simulink model "ModeStEnCtrl6s7s"  (R2024b)
settings: Solver=FixedStepDiscrete  StartTime=0.0  StopTime=10.0  FixedStep=0.01  RelTol=1e-3
undefined symbols (not defined in the file or in its folder): BigFour6sStEnCtrl_Cal, BigFourStEnCtrl_Cal, ComfortMdLStEnCtrl_Cal, ComfortMdRStEnCtrl_Cal, EZE5576sStEnCtrl_Cal, EZE557StEnCtrl_Cal, EZQStEnCtrl_Cal, FirstTrig, INTMLStEnCtrl_Cal, INTMRStEnCtrl_Cal, KeSMSuVehicleModelConfig_Val, LugL6sStEnCtrl_Cal, LugL7sStEnCtrl_Cal, LugR6sStEnCtrl_Cal, LugR7sStEnCtrl_Cal, Md27StEnCtrl_Cal, Md28StEnCtrl_Cal, Md30StEnCtrl_Cal, Md31StEnCtrl_Cal, Md32StEnCtrl_Cal, Md53StEnCtrl_Cal, Md57StEnCtrl_Cal, Md58StEnCtrl_Cal, Md58TrgtPos_Set, Md61StEnCtrl_Cal, Md62StEnCtrl_Cal, RecvR4sStEnCtrl_Cal, VIPL557LTStEnCtrl_Cal, VIPL557StEnCtrl_Cal, VIPLExit557StEnCtrl_Cal, VIPLExit557TrgtPos_Set, VIPR557LTStEnCtrl_Cal, VIPR557StEnCtrl_Cal, VIPRExit557StEnCtrl_Cal, VIPRExit557TrgtPos_Set
libraries: simulink x30
(part 1 of 2)
settings Model: Creator=sn2xws  LastModifiedBy=sn55gm
settings Model: ModifiedHistory=|
  | 2024.5.8
  | V3.0.0 557 eze 及复位模式变更
  | 2024.7.9
  | V3.0.1 557 模式流程V1.9
  | V3.0.2 md30 md31 md32 md53增加mdfirsttrig
  | V3.0.3 md1增加firsttrig
  | V3.0.4 智享增加FirstTrig
  | V3.0.5 Md28 FirstTrig信号遗漏连接
  | V3.0.6 Md27 FirstTrig信号遗漏连接
  | V3.0.7 Md8,Md9增加FirstTrig信号
  | V3.0.8 新增Md56
  | V3.0.9 新增Md57，Md58
  | V3.1.0 BUG 969014 Lug7sRStEnCtrl en 属性改为reset
  | V3.13.0 新增Md61 md62
settings SolverCC: AlgebraicLoopSolver=TrustRegion
settings DataIOCC: SaveFormat=StructureWithTime  ReturnWorkspaceOutputs=off
settings OptimizationCC: DefaultParameterBehavior=Inlined  EnhancedBackFolding=on  PassReuseOutputArgsAs=Individual arguments  ZeroExternalMemoryAtStartup=off  ZeroInternalMemoryAtStartup=off  OptimizeBlockOrder=speed  DifferentSizesBufferReuse=on  OptimizationCustomize=off  EfficientTunableParamExpr=on
settings DebuggingCC: ParameterTunabilityLossMsg=error  UnconnectedInputMsg=warning  UnconnectedOutputMsg=warning  UnconnectedLineMsg=warning  ArithmeticOperatorsInVariantConditions=warning
settings ModelReferenceCC: EnableRefExpFcnMdlSchedulingChecks=on
settings SFSimCC: MATLABDynamicMemAlloc=off  CustomCodeUndefinedFunction=UseInterfaceOnly
settings RTWCC: Description=AUTOSAR  SystemTargetFile=autosar.tlc  GenCodeOnly=on  TemplateMakefile=ert_default_tmf  GenerateReport=on  IncludeHyperlinkInReport=on  LaunchReport=on  DataTypeReplacement=CDataTypesFixedWidth  GenerateTraceInfo=on  GenerateTraceReport=on  GenerateTraceReportSl=on  GenerateTraceReportSf=on  GenerateTraceReportEml=on  GenerateCodeMetricsReport=on  GPUComputeCapability=3.5
settings CodeAppCC: ForceParamTrailComments=on  IgnoreCustomStorageClasses=off  OperatorAnnotations=on  SimulinkDataObjDesc=on  SFDataObjDesc=on  InsertBlockDesc=on
settings STFCustomTargetCC: TargetLangStandard=C99 (ISO)  MultiwordLength=256  ParMdlRefBuildCompliant=on  CompOptLevelCompliant=on  IncludeMdlTerminateFcn=off  CombineOutputUpdateFcns=on  SuppressErrorStatus=on  ERTCustomFileBanners=on  SupportNonFinite=off  SupportComplex=off  SupportContinuousTime=off  SupportNonInlinedSFcns=off  RemoveResetFunc=on  MATLABClassNameForMDSCustomization=Simulink.SoftwareTarget.ERTCustomization  AutosarCompliant=on  UseToolchainInfoCompliant=on  LookupTableObjectStructAxisOrder=2,1,3,4,...  LUTObjectStructOrderEvenSpacing=Size,Table,Breakpoints  SystemTargetFile=autosar.tlc
settings ERTTargetCC: TargetLangStandard=C99 (ISO)  ConcurrentExecutionCompliant=off  IncludeMdlTerminateFcn=off  SuppressErrorStatus=on  SupportNonFinite=off  SupportComplex=off  ModelStepFunctionPrototypeControlCompliant=off  CPPClassGenCompliant=off  AutosarCompliant=on  LookupTableObjectStructAxisOrder=2,1,3,4,...  LUTObjectStructOrderEvenSpacing=Size,Table,Breakpoints  ERTCustomFileTemplate=example_file_process.tlc  ERTFilePackagingFormat=Compact  BooleanTrueId=TRUE  BooleanFalseId=FALSE  DynamicArrayContainerType=coder::array

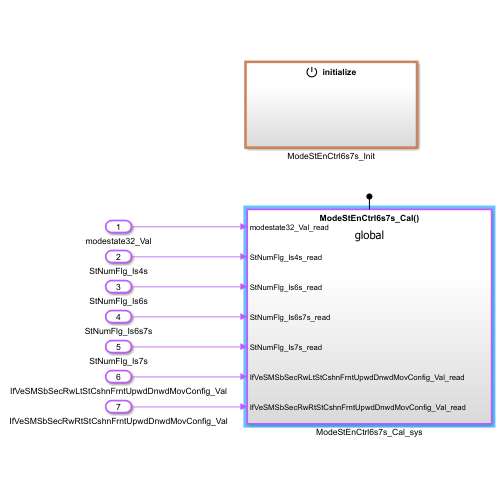
[thumbnail: Simulink's stored preview of the top-level diagram]
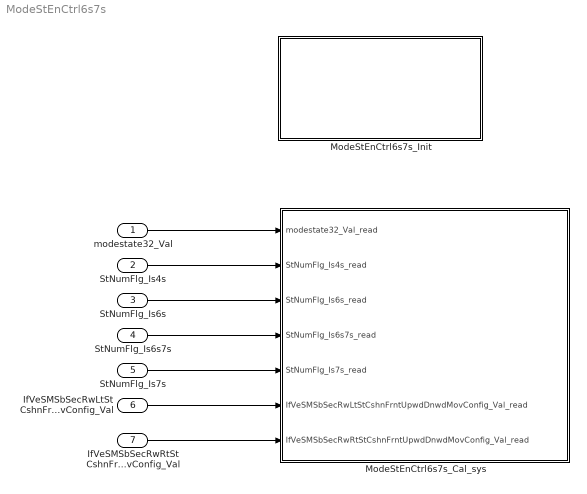
== system ModeStEnCtrl6s7s ==
  modestate32_Val : Inport  OutDataTypeStr=uint32  PortDimensions=1
  StNumFlg_Is4s : Inport  Port=2  OutDataTypeStr=boolean  PortDimensions=1
  StNumFlg_Is6s : Inport  Port=3  OutDataTypeStr=boolean  PortDimensions=1
  StNumFlg_Is6s7s : Inport  Port=4  OutDataTypeStr=boolean  PortDimensions=1
  StNumFlg_Is7s : Inport  Port=5  OutDataTypeStr=boolean  PortDimensions=1
  IfVeSMSbSecRwLtStCshnFrntUpwdDnwdMovConfig_Val : Inport  Port=6  OutDataTypeStr=boolean  PortDimensions=1
  IfVeSMSbSecRwRtStCshnFrntUpwdDnwdMovConfig_Val : Inport  Port=7  OutDataTypeStr=boolean  PortDimensions=1
  ModeStEnCtrl6s7s_Cal_sys : Subsystem
  ModeStEnCtrl6s7s_Init : Subsystem
  wires:
  modestate32_Val/1 -> ModeStEnCtrl6s7s_Cal_sys/1(modestate32_Val_read)
  StNumFlg_Is4s/1 -> ModeStEnCtrl6s7s_Cal_sys/2(StNumFlg_Is4s_read)
  StNumFlg_Is6s/1 -> ModeStEnCtrl6s7s_Cal_sys/3(StNumFlg_Is6s_read)
  StNumFlg_Is6s7s/1 -> ModeStEnCtrl6s7s_Cal_sys/4(StNumFlg_Is6s7s_read)
  StNumFlg_Is7s/1 -> ModeStEnCtrl6s7s_Cal_sys/5(StNumFlg_Is7s_read)
  IfVeSMSbSecRwLtStCshnFrntUpwdDnwdMovConfig_Val/1 -> ModeStEnCtrl6s7s_Cal_sys/6(IfVeSMSbSecRwLtStCshnFrntUpwdDnwdMovConfig_Val_read)
  IfVeSMSbSecRwRtStCshnFrntUpwdDnwdMovConfig_Val/1 -> ModeStEnCtrl6s7s_Cal_sys/7(IfVeSMSbSecRwRtStCshnFrntUpwdDnwdMovConfig_Val_read)

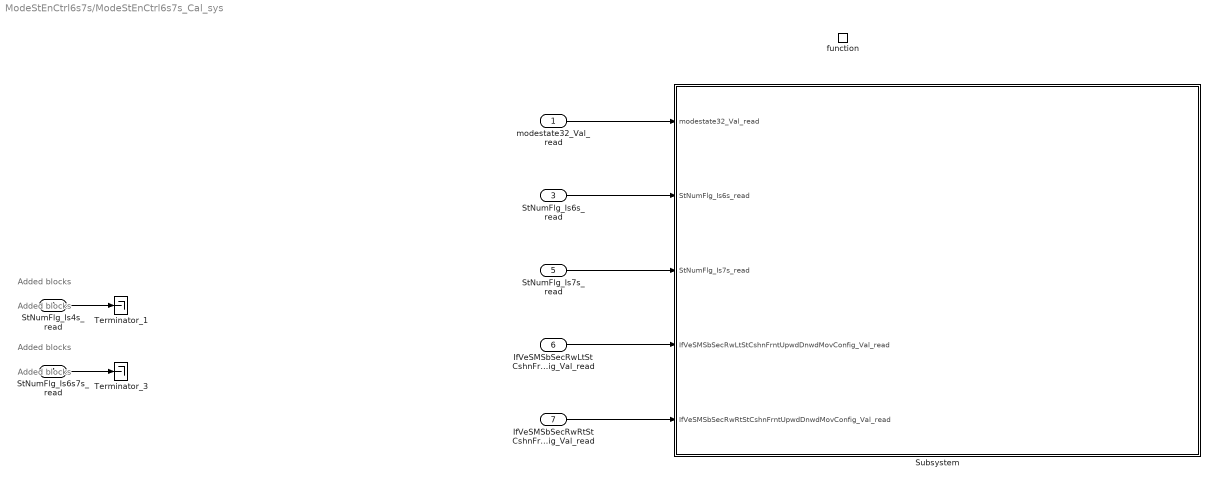
== system ModeStEnCtrl6s7s/ModeStEnCtrl6s7s_Cal_sys ==
  note: Added blocks
  note: Added blocks
  note: Added blocks
  note: Added blocks
  modestate32_Val_read : Inport
  StNumFlg_Is4s_read : Inport  Port=2
  StNumFlg_Is6s_read : Inport  Port=3
  StNumFlg_Is6s7s_read : Inport  Port=4
  StNumFlg_Is7s_read : Inport  Port=5
  IfVeSMSbSecRwLtStCshnFrntUpwdDnwdMovConfig_Val_read : Inport  Port=6
  IfVeSMSbSecRwRtStCshnFrntUpwdDnwdMovConfig_Val_read : Inport  Port=7
  function : TriggerPort  TriggerType=function-call  IsSimulinkFunction=on  FunctionName=ModeStEnCtrl6s7s_Cal  VariantControl=(inherit)
  Subsystem : Subsystem
  Terminator_1 : Terminator
  Terminator_3 : Terminator
  wires:
  modestate32_Val_read/1 -> Subsystem/1(modestate32_Val_read)
  StNumFlg_Is4s_read/1 -> Terminator_1/1
  StNumFlg_Is6s7s_read/1 -> Terminator_3/1
  StNumFlg_Is7s_read/1 -> Subsystem/3(StNumFlg_Is7s_read)
  StNumFlg_Is6s_read/1 -> Subsystem/2(StNumFlg_Is6s_read)
  IfVeSMSbSecRwLtStCshnFrntUpwdDnwdMovConfig_Val_read/1 -> Subsystem/4(IfVeSMSbSecRwLtStCshnFrntUpwdDnwdMovConfig_Val_read)
  IfVeSMSbSecRwRtStCshnFrntUpwdDnwdMovConfig_Val_read/1 -> Subsystem/5(IfVeSMSbSecRwRtStCshnFrntUpwdDnwdMovConfig_Val_read)

== system ModeStEnCtrl6s7s/ModeStEnCtrl6s7s_Init ==
  note: Added blocks
  Event Listener : EventListener  EventName=reset
  PA_KeSMSuVehicleModelConfig_Val : Constant  Value=KeSMSuVehicleModelConfig_Val
  Terminator_1 : Terminator
  wires:
  PA_KeSMSuVehicleModelConfig_Val/1 -> Terminator_1/1

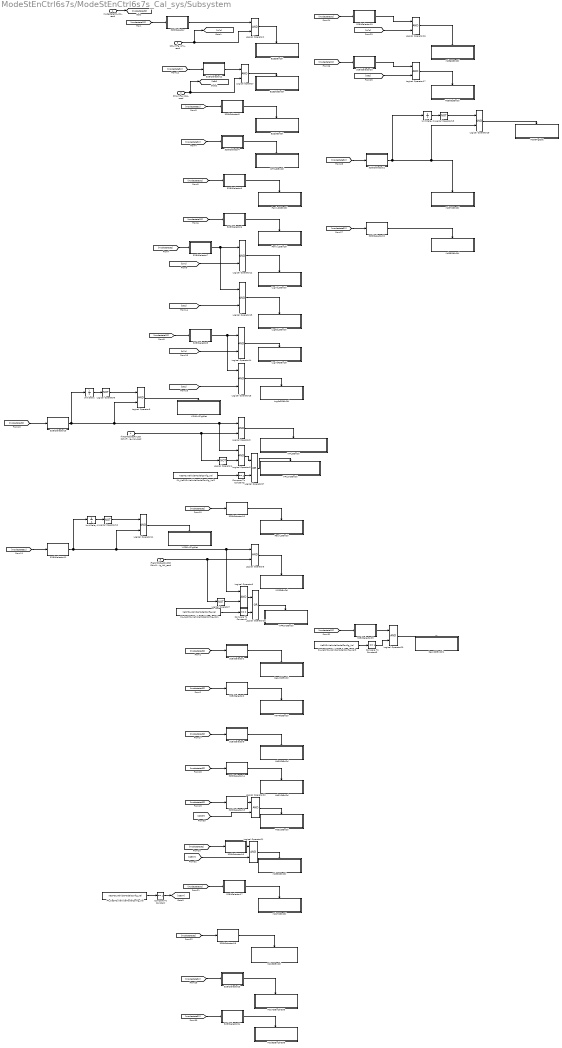
== system ModeStEnCtrl6s7s/ModeStEnCtrl6s7s_Cal_sys/Subsystem ==
  modestate32_Val_read : Inport
  StNumFlg_Is6s_read : Inport  Port=2
  StNumFlg_Is7s_read : Inport  Port=3
  IfVeSMSbSecRwLtStCshnFrntUpwdDnwdMovConfig_Val_read : Inport  Port=4
  IfVeSMSbSecRwRtStCshnFrntUpwdDnwdMovConfig_Val_read : Inport  Port=5
  32BitSelector : Subsystem  mask(32 Bit Selector){BitNum=0}
      mask prompts: BitNum "Select Bit Number"
      mask help: Allows selection of a particular bit (0-31) out of a packed word up to 32 bits long. Output will be true if the bit number selected via the mask parameter is equal to one.
      mask TypeOptions BitNum: 0 | 1 | 2 | 3 | 4 | 5 | 6 | 7 | 8 | 9 | 10 | 11 | 12 | 13 | 14 | 15 | 16 | 17 | 18 | 19 | 20 | 21 | 22 | 23 | 24 | 25 | 26 | 27 | 28 | 29 | 30 | 31
      mask Display:
      | text(0.5, 0.8,'BIT','horizontalAlignment','center')
      | text(0.5, 0.5,'SELECTOR','horizontalAlignment','center')
      | text(0.5, 0.2,['-- Bit ',char(get_param(gcb,'BitNum')),' --'],'horizontalAlignment','center')
  32BitSelector1 : Subsystem  mask(32 Bit Selector){BitNum=12}
      mask prompts: BitNum "Select Bit Number"
      mask help: Allows selection of a particular bit (0-31) out of a packed word up to 32 bits long. Output will be true if the bit number selected via the mask parameter is equal to one.
      mask TypeOptions BitNum: 0 | 1 | 2 | 3 | 4 | 5 | 6 | 7 | 8 | 9 | 10 | 11 | 12 | 13 | 14 | 15 | 16 | 17 | 18 | 19 | 20 | 21 | 22 | 23 | 24 | 25 | 26 | 27 | 28 | 29 | 30 | 31
      mask Display:
      | text(0.5, 0.8,'BIT','horizontalAlignment','center')
      | text(0.5, 0.5,'SELECTOR','horizontalAlignment','center')
      | text(0.5, 0.2,['-- Bit ',char(get_param(gcb,'BitNum')),' --'],'horizontalAlignment','center')
  32BitSelector10 : Subsystem  mask(32 Bit Selector){BitNum=10}
      mask prompts: BitNum "Select Bit Number"
      mask help: Allows selection of a particular bit (0-31) out of a packed word up to 32 bits long. Output will be true if the bit number selected via the mask parameter is equal to one.
      mask TypeOptions BitNum: 0 | 1 | 2 | 3 | 4 | 5 | 6 | 7 | 8 | 9 | 10 | 11 | 12 | 13 | 14 | 15 | 16 | 17 | 18 | 19 | 20 | 21 | 22 | 23 | 24 | 25 | 26 | 27 | 28 | 29 | 30 | 31
      mask Display:
      | text(0.5, 0.8,'BIT','horizontalAlignment','center')
      | text(0.5, 0.5,'SELECTOR','horizontalAlignment','center')
      | text(0.5, 0.2,['-- Bit ',char(get_param(gcb,'BitNum')),' --'],'horizontalAlignment','center')
  32BitSelector11 : Subsystem  mask(32 Bit Selector){BitNum=11}
      mask prompts: BitNum "Select Bit Number"
      mask help: Allows selection of a particular bit (0-31) out of a packed word up to 32 bits long. Output will be true if the bit number selected via the mask parameter is equal to one.
      mask TypeOptions BitNum: 0 | 1 | 2 | 3 | 4 | 5 | 6 | 7 | 8 | 9 | 10 | 11 | 12 | 13 | 14 | 15 | 16 | 17 | 18 | 19 | 20 | 21 | 22 | 23 | 24 | 25 | 26 | 27 | 28 | 29 | 30 | 31
      mask Display:
      | text(0.5, 0.8,'BIT','horizontalAlignment','center')
      | text(0.5, 0.5,'SELECTOR','horizontalAlignment','center')
      | text(0.5, 0.2,['-- Bit ',char(get_param(gcb,'BitNum')),' --'],'horizontalAlignment','center')
  32BitSelector12 : Subsystem  mask(32 Bit Selector){BitNum=0}
      mask prompts: BitNum "Select Bit Number"
      mask help: Allows selection of a particular bit (0-31) out of a packed word up to 32 bits long. Output will be true if the bit number selected via the mask parameter is equal to one.
      mask TypeOptions BitNum: 0 | 1 | 2 | 3 | 4 | 5 | 6 | 7 | 8 | 9 | 10 | 11 | 12 | 13 | 14 | 15 | 16 | 17 | 18 | 19 | 20 | 21 | 22 | 23 | 24 | 25 | 26 | 27 | 28 | 29 | 30 | 31
      mask Display:
      | text(0.5, 0.8,'BIT','horizontalAlignment','center')
      | text(0.5, 0.5,'SELECTOR','horizontalAlignment','center')
      | text(0.5, 0.2,['-- Bit ',char(get_param(gcb,'BitNum')),' --'],'horizontalAlignment','center')
  32BitSelector13 : Subsystem  mask(32 Bit Selector){BitNum=9}
      mask prompts: BitNum "Select Bit Number"
      mask help: Allows selection of a particular bit (0-31) out of a packed word up to 32 bits long. Output will be true if the bit number selected via the mask parameter is equal to one.
      mask TypeOptions BitNum: 0 | 1 | 2 | 3 | 4 | 5 | 6 | 7 | 8 | 9 | 10 | 11 | 12 | 13 | 14 | 15 | 16 | 17 | 18 | 19 | 20 | 21 | 22 | 23 | 24 | 25 | 26 | 27 | 28 | 29 | 30 | 31
      mask Display:
      | text(0.5, 0.8,'BIT','horizontalAlignment','center')
      | text(0.5, 0.5,'SELECTOR','horizontalAlignment','center')
      | text(0.5, 0.2,['-- Bit ',char(get_param(gcb,'BitNum')),' --'],'horizontalAlignment','center')
  32BitSelector14 : Subsystem  mask(32 Bit Selector){BitNum=30}
      mask prompts: BitNum "Select Bit Number"
      mask help: Allows selection of a particular bit (0-31) out of a packed word up to 32 bits long. Output will be true if the bit number selected via the mask parameter is equal to one.
      mask TypeOptions BitNum: 0 | 1 | 2 | 3 | 4 | 5 | 6 | 7 | 8 | 9 | 10 | 11 | 12 | 13 | 14 | 15 | 16 | 17 | 18 | 19 | 20 | 21 | 22 | 23 | 24 | 25 | 26 | 27 | 28 | 29 | 30 | 31
      mask Display:
      | text(0.5, 0.8,'BIT','horizontalAlignment','center')
      | text(0.5, 0.5,'SELECTOR','horizontalAlignment','center')
      | text(0.5, 0.2,['-- Bit ',char(get_param(gcb,'BitNum')),' --'],'horizontalAlignment','center')
  32BitSelector15 : Subsystem  mask(32 Bit Selector){BitNum=31}
      mask prompts: BitNum "Select Bit Number"
      mask help: Allows selection of a particular bit (0-31) out of a packed word up to 32 bits long. Output will be true if the bit number selected via the mask parameter is equal to one.
      mask TypeOptions BitNum: 0 | 1 | 2 | 3 | 4 | 5 | 6 | 7 | 8 | 9 | 10 | 11 | 12 | 13 | 14 | 15 | 16 | 17 | 18 | 19 | 20 | 21 | 22 | 23 | 24 | 25 | 26 | 27 | 28 | 29 | 30 | 31
      mask Display:
      | text(0.5, 0.8,'BIT','horizontalAlignment','center')
      | text(0.5, 0.5,'SELECTOR','horizontalAlignment','center')
      | text(0.5, 0.2,['-- Bit ',char(get_param(gcb,'BitNum')),' --'],'horizontalAlignment','center')
  32BitSelector16 : Subsystem  mask(32 Bit Selector){BitNum=17}
      mask prompts: BitNum "Select Bit Number"
      mask help: Allows selection of a particular bit (0-31) out of a packed word up to 32 bits long. Output will be true if the bit number selected via the mask parameter is equal to one.
      mask TypeOptions BitNum: 0 | 1 | 2 | 3 | 4 | 5 | 6 | 7 | 8 | 9 | 10 | 11 | 12 | 13 | 14 | 15 | 16 | 17 | 18 | 19 | 20 | 21 | 22 | 23 | 24 | 25 | 26 | 27 | 28 | 29 | 30 | 31
      mask Display:
      | text(0.5, 0.8,'BIT','horizontalAlignment','center')
      | text(0.5, 0.5,'SELECTOR','horizontalAlignment','center')
      | text(0.5, 0.2,['-- Bit ',char(get_param(gcb,'BitNum')),' --'],'horizontalAlignment','center')
  32BitSelector17 : Subsystem  mask(32 Bit Selector){BitNum=26}
      mask prompts: BitNum "Select Bit Number"
      mask help: Allows selection of a particular bit (0-31) out of a packed word up to 32 bits long. Output will be true if the bit number selected via the mask parameter is equal to one.
      mask TypeOptions BitNum: 0 | 1 | 2 | 3 | 4 | 5 | 6 | 7 | 8 | 9 | 10 | 11 | 12 | 13 | 14 | 15 | 16 | 17 | 18 | 19 | 20 | 21 | 22 | 23 | 24 | 25 | 26 | 27 | 28 | 29 | 30 | 31
      mask Display:
      | text(0.5, 0.8,'BIT','horizontalAlignment','center')
      | text(0.5, 0.5,'SELECTOR','horizontalAlignment','center')
      | text(0.5, 0.2,['-- Bit ',char(get_param(gcb,'BitNum')),' --'],'horizontalAlignment','center')
  32BitSelector18 : Subsystem  mask(32 Bit Selector){BitNum=27}
      mask prompts: BitNum "Select Bit Number"
      mask help: Allows selection of a particular bit (0-31) out of a packed word up to 32 bits long. Output will be true if the bit number selected via the mask parameter is equal to one.
      mask TypeOptions BitNum: 0 | 1 | 2 | 3 | 4 | 5 | 6 | 7 | 8 | 9 | 10 | 11 | 12 | 13 | 14 | 15 | 16 | 17 | 18 | 19 | 20 | 21 | 22 | 23 | 24 | 25 | 26 | 27 | 28 | 29 | 30 | 31
      mask Display:
      | text(0.5, 0.8,'BIT','horizontalAlignment','center')
      | text(0.5, 0.5,'SELECTOR','horizontalAlignment','center')
      | text(0.5, 0.2,['-- Bit ',char(get_param(gcb,'BitNum')),' --'],'horizontalAlignment','center')
  32BitSelector19 : Subsystem  mask(32 Bit Selector){BitNum=24}
      mask prompts: BitNum "Select Bit Number"
      mask help: Allows selection of a particular bit (0-31) out of a packed word up to 32 bits long. Output will be true if the bit number selected via the mask parameter is equal to one.
      mask TypeOptions BitNum: 0 | 1 | 2 | 3 | 4 | 5 | 6 | 7 | 8 | 9 | 10 | 11 | 12 | 13 | 14 | 15 | 16 | 17 | 18 | 19 | 20 | 21 | 22 | 23 | 24 | 25 | 26 | 27 | 28 | 29 | 30 | 31
      mask Display:
      | text(0.5, 0.8,'BIT','horizontalAlignment','center')
      | text(0.5, 0.5,'SELECTOR','horizontalAlignment','center')
      | text(0.5, 0.2,['-- Bit ',char(get_param(gcb,'BitNum')),' --'],'horizontalAlignment','center')
  32BitSelector2 : Subsystem  mask(32 Bit Selector){BitNum=19}
      mask prompts: BitNum "Select Bit Number"
      mask help: Allows selection of a particular bit (0-31) out of a packed word up to 32 bits long. Output will be true if the bit number selected via the mask parameter is equal to one.
      mask TypeOptions BitNum: 0 | 1 | 2 | 3 | 4 | 5 | 6 | 7 | 8 | 9 | 10 | 11 | 12 | 13 | 14 | 15 | 16 | 17 | 18 | 19 | 20 | 21 | 22 | 23 | 24 | 25 | 26 | 27 | 28 | 29 | 30 | 31
      mask Display:
      | text(0.5, 0.8,'BIT','horizontalAlignment','center')
      | text(0.5, 0.5,'SELECTOR','horizontalAlignment','center')
      | text(0.5, 0.2,['-- Bit ',char(get_param(gcb,'BitNum')),' --'],'horizontalAlignment','center')
  32BitSelector20 : Subsystem  mask(32 Bit Selector){BitNum=24}
      mask prompts: BitNum "Select Bit Number"
      mask help: Allows selection of a particular bit (0-31) out of a packed word up to 32 bits long. Output will be true if the bit number selected via the mask parameter is equal to one.
      mask TypeOptions BitNum: 0 | 1 | 2 | 3 | 4 | 5 | 6 | 7 | 8 | 9 | 10 | 11 | 12 | 13 | 14 | 15 | 16 | 17 | 18 | 19 | 20 | 21 | 22 | 23 | 24 | 25 | 26 | 27 | 28 | 29 | 30 | 31
      mask Display:
      | text(0.5, 0.8,'BIT','horizontalAlignment','center')
      | text(0.5, 0.5,'SELECTOR','horizontalAlignment','center')
      | text(0.5, 0.2,['-- Bit ',char(get_param(gcb,'BitNum')),' --'],'horizontalAlignment','center')
  32BitSelector21 : Subsystem  mask(32 Bit Selector){BitNum=20}
      mask prompts: BitNum "Select Bit Number"
      mask help: Allows selection of a particular bit (0-31) out of a packed word up to 32 bits long. Output will be true if the bit number selected via the mask parameter is equal to one.
      mask TypeOptions BitNum: 0 | 1 | 2 | 3 | 4 | 5 | 6 | 7 | 8 | 9 | 10 | 11 | 12 | 13 | 14 | 15 | 16 | 17 | 18 | 19 | 20 | 21 | 22 | 23 | 24 | 25 | 26 | 27 | 28 | 29 | 30 | 31
      mask Display:
      | text(0.5, 0.8,'BIT','horizontalAlignment','center')
      | text(0.5, 0.5,'SELECTOR','horizontalAlignment','center')
      | text(0.5, 0.2,['-- Bit ',char(get_param(gcb,'BitNum')),' --'],'horizontalAlignment','center')
  32BitSelector22 : Subsystem  mask(32 Bit Selector){BitNum=21}
      mask prompts: BitNum "Select Bit Number"
      mask help: Allows selection of a particular bit (0-31) out of a packed word up to 32 bits long. Output will be true if the bit number selected via the mask parameter is equal to one.
      mask TypeOptions BitNum: 0 | 1 | 2 | 3 | 4 | 5 | 6 | 7 | 8 | 9 | 10 | 11 | 12 | 13 | 14 | 15 | 16 | 17 | 18 | 19 | 20 | 21 | 22 | 23 | 24 | 25 | 26 | 27 | 28 | 29 | 30 | 31
      mask Display:
      | text(0.5, 0.8,'BIT','horizontalAlignment','center')
      | text(0.5, 0.5,'SELECTOR','horizontalAlignment','center')
      | text(0.5, 0.2,['-- Bit ',char(get_param(gcb,'BitNum')),' --'],'horizontalAlignment','center')
  32BitSelector23 : Subsystem  mask(32 Bit Selector){BitNum=13}
      mask prompts: BitNum "Select Bit Number"
      mask help: Allows selection of a particular bit (0-31) out of a packed word up to 32 bits long. Output will be true if the bit number selected via the mask parameter is equal to one.
      mask TypeOptions BitNum: 0 | 1 | 2 | 3 | 4 | 5 | 6 | 7 | 8 | 9 | 10 | 11 | 12 | 13 | 14 | 15 | 16 | 17 | 18 | 19 | 20 | 21 | 22 | 23 | 24 | 25 | 26 | 27 | 28 | 29 | 30 | 31
      mask Display:
      | text(0.5, 0.8,'BIT','horizontalAlignment','center')
      | text(0.5, 0.5,'SELECTOR','horizontalAlignment','center')
      | text(0.5, 0.2,['-- Bit ',char(get_param(gcb,'BitNum')),' --'],'horizontalAlignment','center')
  32BitSelector24 : Subsystem  mask(32 Bit Selector){BitNum=14}
      mask prompts: BitNum "Select Bit Number"
      mask help: Allows selection of a particular bit (0-31) out of a packed word up to 32 bits long. Output will be true if the bit number selected via the mask parameter is equal to one.
      mask TypeOptions BitNum: 0 | 1 | 2 | 3 | 4 | 5 | 6 | 7 | 8 | 9 | 10 | 11 | 12 | 13 | 14 | 15 | 16 | 17 | 18 | 19 | 20 | 21 | 22 | 23 | 24 | 25 | 26 | 27 | 28 | 29 | 30 | 31
      mask Display:
      | text(0.5, 0.8,'BIT','horizontalAlignment','center')
      | text(0.5, 0.5,'SELECTOR','horizontalAlignment','center')
      | text(0.5, 0.2,['-- Bit ',char(get_param(gcb,'BitNum')),' --'],'horizontalAlignment','center')
  32BitSelector25 : Subsystem  mask(32 Bit Selector){BitNum=12}
      mask prompts: BitNum "Select Bit Number"
      mask help: Allows selection of a particular bit (0-31) out of a packed word up to 32 bits long. Output will be true if the bit number selected via the mask parameter is equal to one.
      mask TypeOptions BitNum: 0 | 1 | 2 | 3 | 4 | 5 | 6 | 7 | 8 | 9 | 10 | 11 | 12 | 13 | 14 | 15 | 16 | 17 | 18 | 19 | 20 | 21 | 22 | 23 | 24 | 25 | 26 | 27 | 28 | 29 | 30 | 31
      mask Display:
      | text(0.5, 0.8,'BIT','horizontalAlignment','center')
      | text(0.5, 0.5,'SELECTOR','horizontalAlignment','center')
      | text(0.5, 0.2,['-- Bit ',char(get_param(gcb,'BitNum')),' --'],'horizontalAlignment','center')
  32BitSelector3 : Subsystem  mask(32 Bit Selector){BitNum=3}
      mask prompts: BitNum "Select Bit Number"
      mask help: Allows selection of a particular bit (0-31) out of a packed word up to 32 bits long. Output will be true if the bit number selected via the mask parameter is equal to one.
      mask TypeOptions BitNum: 0 | 1 | 2 | 3 | 4 | 5 | 6 | 7 | 8 | 9 | 10 | 11 | 12 | 13 | 14 | 15 | 16 | 17 | 18 | 19 | 20 | 21 | 22 | 23 | 24 | 25 | 26 | 27 | 28 | 29 | 30 | 31
      mask Display:
      | text(0.5, 0.8,'BIT','horizontalAlignment','center')
      | text(0.5, 0.5,'SELECTOR','horizontalAlignment','center')
      | text(0.5, 0.2,['-- Bit ',char(get_param(gcb,'BitNum')),' --'],'horizontalAlignment','center')
  32BitSelector4 : Subsystem  mask(32 Bit Selector){BitNum=4}
      mask prompts: BitNum "Select Bit Number"
      mask help: Allows selection of a particular bit (0-31) out of a packed word up to 32 bits long. Output will be true if the bit number selected via the mask parameter is equal to one.
      mask TypeOptions BitNum: 0 | 1 | 2 | 3 | 4 | 5 | 6 | 7 | 8 | 9 | 10 | 11 | 12 | 13 | 14 | 15 | 16 | 17 | 18 | 19 | 20 | 21 | 22 | 23 | 24 | 25 | 26 | 27 | 28 | 29 | 30 | 31
      mask Display:
      | text(0.5, 0.8,'BIT','horizontalAlignment','center')
      | text(0.5, 0.5,'SELECTOR','horizontalAlignment','center')
      | text(0.5, 0.2,['-- Bit ',char(get_param(gcb,'BitNum')),' --'],'horizontalAlignment','center')
  32BitSelector5 : Subsystem  mask(32 Bit Selector){BitNum=5}
      mask prompts: BitNum "Select Bit Number"
      mask help: Allows selection of a particular bit (0-31) out of a packed word up to 32 bits long. Output will be true if the bit number selected via the mask parameter is equal to one.
      mask TypeOptions BitNum: 0 | 1 | 2 | 3 | 4 | 5 | 6 | 7 | 8 | 9 | 10 | 11 | 12 | 13 | 14 | 15 | 16 | 17 | 18 | 19 | 20 | 21 | 22 | 23 | 24 | 25 | 26 | 27 | 28 | 29 | 30 | 31
      mask Display:
      | text(0.5, 0.8,'BIT','horizontalAlignment','center')
      | text(0.5, 0.5,'SELECTOR','horizontalAlignment','center')
      | text(0.5, 0.2,['-- Bit ',char(get_param(gcb,'BitNum')),' --'],'horizontalAlignment','center')
  32BitSelector6 : Subsystem  mask(32 Bit Selector){BitNum=6}
      mask prompts: BitNum "Select Bit Number"
      mask help: Allows selection of a particular bit (0-31) out of a packed word up to 32 bits long. Output will be true if the bit number selected via the mask parameter is equal to one.
      mask TypeOptions BitNum: 0 | 1 | 2 | 3 | 4 | 5 | 6 | 7 | 8 | 9 | 10 | 11 | 12 | 13 | 14 | 15 | 16 | 17 | 18 | 19 | 20 | 21 | 22 | 23 | 24 | 25 | 26 | 27 | 28 | 29 | 30 | 31
      mask Display:
      | text(0.5, 0.8,'BIT','horizontalAlignment','center')
      | text(0.5, 0.5,'SELECTOR','horizontalAlignment','center')
      | text(0.5, 0.2,['-- Bit ',char(get_param(gcb,'BitNum')),' --'],'horizontalAlignment','center')
  32BitSelector7 : Subsystem  mask(32 Bit Selector){BitNum=7}
      mask prompts: BitNum "Select Bit Number"
      mask help: Allows selection of a particular bit (0-31) out of a packed word up to 32 bits long. Output will be true if the bit number selected via the mask parameter is equal to one.
      mask TypeOptions BitNum: 0 | 1 | 2 | 3 | 4 | 5 | 6 | 7 | 8 | 9 | 10 | 11 | 12 | 13 | 14 | 15 | 16 | 17 | 18 | 19 | 20 | 21 | 22 | 23 | 24 | 25 | 26 | 27 | 28 | 29 | 30 | 31
      mask Display:
      | text(0.5, 0.8,'BIT','horizontalAlignment','center')
      | text(0.5, 0.5,'SELECTOR','horizontalAlignment','center')
      | text(0.5, 0.2,['-- Bit ',char(get_param(gcb,'BitNum')),' --'],'horizontalAlignment','center')
  32BitSelector8 : Subsystem  mask(32 Bit Selector){BitNum=8}
      mask prompts: BitNum "Select Bit Number"
      mask help: Allows selection of a particular bit (0-31) out of a packed word up to 32 bits long. Output will be true if the bit number selected via the mask parameter is equal to one.
      mask TypeOptions BitNum: 0 | 1 | 2 | 3 | 4 | 5 | 6 | 7 | 8 | 9 | 10 | 11 | 12 | 13 | 14 | 15 | 16 | 17 | 18 | 19 | 20 | 21 | 22 | 23 | 24 | 25 | 26 | 27 | 28 | 29 | 30 | 31
      mask Display:
      | text(0.5, 0.8,'BIT','horizontalAlignment','center')
      | text(0.5, 0.5,'SELECTOR','horizontalAlignment','center')
      | text(0.5, 0.2,['-- Bit ',char(get_param(gcb,'BitNum')),' --'],'horizontalAlignment','center')
  32BitSelector9 : Subsystem  mask(32 Bit Selector){BitNum=29}
      mask prompts: BitNum "Select Bit Number"
      mask help: Allows selection of a particular bit (0-31) out of a packed word up to 32 bits long. Output will be true if the bit number selected via the mask parameter is equal to one.
      mask TypeOptions BitNum: 0 | 1 | 2 | 3 | 4 | 5 | 6 | 7 | 8 | 9 | 10 | 11 | 12 | 13 | 14 | 15 | 16 | 17 | 18 | 19 | 20 | 21 | 22 | 23 | 24 | 25 | 26 | 27 | 28 | 29 | 30 | 31
      mask Display:
      | text(0.5, 0.8,'BIT','horizontalAlignment','center')
      | text(0.5, 0.5,'SELECTOR','horizontalAlignment','center')
      | text(0.5, 0.2,['-- Bit ',char(get_param(gcb,'BitNum')),' --'],'horizontalAlignment','center')
  Compare To Constant : simulink/Logic and Bit Operations/Compare To Constant  relop===  const=1  OutDataTypeStr=boolean
  Compare To Constant1 : simulink/Logic and Bit Operations/Compare To Constant  relop===  const=2  OutDataTypeStr=boolean
  Compare To Constant2 : simulink/Logic and Bit Operations/Compare To Constant  relop===  const=2  OutDataTypeStr=boolean
  Compare To Constant3 : simulink/Logic and Bit Operations/Compare To Constant  relop===  const=1  OutDataTypeStr=boolean
  EZES6stEnCtrl : Subsystem  TreatAsAtomicUnit=on
  EZEStEnCtrl : Subsystem  TreatAsAtomicUnit=on
  EZQStEnCtrl : Subsystem  TreatAsAtomicUnit=on
  FamlyLStEnCtrl : Subsystem  TreatAsAtomicUnit=on
  FamlyRStEnCtrl : Subsystem  TreatAsAtomicUnit=on
  INTMLStEnCtrl : Subsystem  TreatAsAtomicUnit=on
  INTMRStEnCtrl : Subsystem  TreatAsAtomicUnit=on
  Logical Operator{,1..3,5..6,9,11..17,19..22} (18 alike) : Logic  AllPortsSameDT=off  OutDataTypeStr=boolean
  Logical Operator{4,7..8,10,18} (5 alike) : Logic  Operator=NOT  AllPortsSameDT=off  OutDataTypeStr=boolean
  Logical Operator26 : Logic  Operator=OR  AllPortsSameDT=off  OutDataTypeStr=boolean
  Logical Operator27 : Logic  Operator=OR  AllPortsSameDT=off  OutDataTypeStr=boolean
  Lug6sLStEnCtrl : Subsystem  TreatAsAtomicUnit=on
  Lug6sRStEnCtrl : Subsystem  TreatAsAtomicUnit=on
  Lug7sLStEnCtrl : Subsystem  TreatAsAtomicUnit=on
  Lug7sRStEnCtrl : Subsystem  TreatAsAtomicUnit=on
  Md27StEnCtrl : Subsystem  TreatAsAtomicUnit=on
  "Md27StEnCtrl358 " : Subsystem  TreatAsAtomicUnit=on
  Md28StEnCtrl : Subsystem  TreatAsAtomicUnit=on
  "Md28StEnCtrl358 " : Subsystem  TreatAsAtomicUnit=on
  Md30StEnCtrl : Subsystem  TreatAsAtomicUnit=on
  Md31StEnCtrl : Subsystem  TreatAsAtomicUnit=on
  Md32StEnCtrl : Subsystem  TreatAsAtomicUnit=on
  Md53StEnCtrl : Subsystem  TreatAsAtomicUnit=on
  Md566stEnCtrl : Subsystem  TreatAsAtomicUnit=on
  Md56StEnCtrl : Subsystem  TreatAsAtomicUnit=on
  Md57StEnCtrl : Subsystem  TreatAsAtomicUnit=on
  Md58StEnCtrl : Subsystem  TreatAsAtomicUnit=on
  Md58TrgtSet : Subsystem  TreatAsAtomicUnit=on
  PA_KeSMSuVehicleModelConfig_Val{,1..3} (4 alike) : Constant  Value=KeSMSuVehicleModelConfig_Val
  RecvLStEnCtrl : Subsystem  TreatAsAtomicUnit=on
  RecvRStEnCtrl : Subsystem  TreatAsAtomicUnit=on
  RecvRStEnCtrl1 : Subsystem  TreatAsAtomicUnit=on
  Unit Delay : UnitDelay  SampleTime=-1  HasFrameUpgradeWarning=on
  Unit Delay1 : UnitDelay  SampleTime=-1  HasFrameUpgradeWarning=on
  Unit Delay2 : UnitDelay  SampleTime=-1  HasFrameUpgradeWarning=on
  VIPLExitTrgtSet : Subsystem  TreatAsAtomicUnit=on
  VIPLLTStEnCtrl : Subsystem  TreatAsAtomicUnit=on
  VIPLStEnCtrl : Subsystem  TreatAsAtomicUnit=on
  VIPRExitTrgtSet : Subsystem  TreatAsAtomicUnit=on
  VIPRLTStEnCtrl : Subsystem  TreatAsAtomicUnit=on
  VIPRStEnCtrl : Subsystem  TreatAsAtomicUnit=on
  wires:
  32BitSelector5/1(y) -> FamlyRStEnCtrl/Enable
  32BitSelector10/1(y) -> RecvLStEnCtrl/Enable
  [modestate32] -> 32BitSelector1/1(x)
  32BitSelector1/1(y) -> RecvRStEnCtrl/Enable
  [modestate32] -> 32BitSelector10/1(x)
  32BitSelector3/1(y) -> EZQStEnCtrl/Enable
  [modestate32] -> 32BitSelector/1(x)
  [modestate32] -> 32BitSelector11/1(x)
  [modestate32] -> 32BitSelector8/1(x)
  [modestate32] -> 32BitSelector6/1(x)
  32BitSelector6/1(y) -> FamlyLStEnCtrl/Enable
  [modestate32] -> 32BitSelector5/1(x)
  [modestate32] -> 32BitSelector3/1(x)
  [modestate32] -> 32BitSelector4/1(x)
  32BitSelector4/1(y) -> INTMLStEnCtrl/Enable
  [modestate32] -> 32BitSelector7/1(x)
  [modestate32] -> 32BitSelector2/1(x)
  modestate32_Val_read/1 -> [modestate32]
  [modestate32] -> 32BitSelector12/1(x)
  32BitSelector12/1(y) -> Logical Operator/1
  StNumFlg_Is6s_read/1 -> [Is6s], Logical Operator/2
  Logical Operator/1 -> EZES6stEnCtrl/Enable
  32BitSelector/1(y) -> Logical Operator1/1
  Logical Operator1/1 -> EZEStEnCtrl/Enable
  StNumFlg_Is7s_read/1 -> [Is7s], Logical Operator1/2
  [modestate32] -> 32BitSelector13/1(x)
  IfVeSMSbSecRwLtStCshnFrntUpwdDnwdMovConfig_Val_read/1 -> Logical Operator4/1, Logical Operator2/2
  Logical Operator2/1 -> VIPLStEnCtrl/Enable
  Logical Operator4/1 -> Logical Operator3/2
  Logical Operator5/1 -> VIPRStEnCtrl/Enable
  IfVeSMSbSecRwRtStCshnFrntUpwdDnwdMovConfig_Val_read/1 -> Logical Operator7/1, Logical Operator5/2
  Logical Operator7/1 -> Logical Operator6/2
  32BitSelector13/1(y) -> Unit Delay/1, Logical Operator9/2, Logical Operator3/1, Logical Operator2/1
  Unit Delay/1 -> Logical Operator8/1
  Logical Operator8/1 -> Logical Operator9/1
  Logical Operator9/1 -> VIPLExitTrgtSet/Enable
  Logical Operator11/1 -> VIPRExitTrgtSet/Enable
  Logical Operator10/1 -> Logical Operator11/1
  Unit Delay1/1 -> Logical Operator10/1
  32BitSelector11/1(y) -> Unit Delay1/1, Logical Operator11/2, Logical Operator6/1, Logical Operator5/1
  32BitSelector2/1(y) -> INTMRStEnCtrl/Enable
  [Is7s] -> Logical Operator12/2
  Logical Operator12/1 -> Lug7sLStEnCtrl/Enable
  32BitSelector7/1(y) -> Logical Operator13/1, Logical Operator12/1
  [Is6s] -> Logical Operator13/2
  Logical Operator13/1 -> Lug6sLStEnCtrl/Enable
  32BitSelector8/1(y) -> Logical Operator15/1, Logical Operator14/1
  Logical Operator14/1 -> Lug7sRStEnCtrl/Enable
  [Is7s] -> Logical Operator14/2
  [Is6s] -> Logical Operator15/2
  Logical Operator15/1 -> Lug6sRStEnCtrl/Enable
  32BitSelector9/1(y) -> Md30StEnCtrl/Enable
  [modestate32] -> 32BitSelector9/1(x)
  [modestate32] -> 32BitSelector14/1(x)
  32BitSelector14/1(y) -> Md31StEnCtrl/Enable
  [modestate32] -> 32BitSelector15/1(x)
  [modestate32] -> 32BitSelector16/1(x)
  [modestate32] -> 32BitSelector17/1(x)
  [modestate32] -> 32BitSelector18/1(x)
  [Is7s] -> Logical Operator16/2
  Logical Operator16/1 -> Md56StEnCtrl/Enable
  32BitSelector19/1(y) -> Logical Operator16/1
  [modestate32] -> 32BitSelector19/1(x)
  [modestate32] -> 32BitSelector20/1(x)
  32BitSelector20/1(y) -> Logical Operator17/1
  [Is6s] -> Logical Operator17/2
  Logical Operator17/1 -> Md566stEnCtrl/Enable
  [modestate32] -> 32BitSelector21/1(x)
  32BitSelector22/1(y) -> Md58StEnCtrl/Enable
  [modestate32] -> 32BitSelector22/1(x)
  Unit Delay2/1 -> Logical Operator18/1
  32BitSelector21/1(y) -> Unit Delay2/1, Logical Operator19/2, Md57StEnCtrl/Enable
  Logical Operator19/1 -> Md58TrgtSet/Enable
  Logical Operator18/1 -> Logical Operator19/1
  32BitSelector17/1(y) -> Md27StEnCtrl/Enable
  PA_KeSMSuVehicleModelConfig_Val/1 -> Compare To Constant/1
  Compare To Constant/1 -> [IS557]
  PA_KeSMSuVehicleModelConfig_Val1/1 -> Compare To Constant1/1
  Logical Operator6/1 -> Logical Operator26/1
  Compare To Constant1/1 -> Logical Operator26/2
  Logical Operator26/1 -> VIPRLTStEnCtrl/Enable
  Compare To Constant2/1 -> Logical Operator27/2
  PA_KeSMSuVehicleModelConfig_Val2/1 -> Compare To Constant2/1
  Logical Operator3/1 -> Logical Operator27/1
  Logical Operator27/1 -> VIPLLTStEnCtrl/Enable
  32BitSelector18/1(y) -> Md28StEnCtrl/Enable
  [modestate32] -> 32BitSelector23/1(x)
  32BitSelector23/1(y) -> "Md27StEnCtrl358 "/Enable
  [modestate32] -> 32BitSelector24/1(x)
  32BitSelector24/1(y) -> "Md28StEnCtrl358 "/Enable
  PA_KeSMSuVehicleModelConfig_Val3/1 -> Compare To Constant3/1
  [modestate32] -> 32BitSelector25/1(x)
  32BitSelector25/1(y) -> Logical Operator20/1
  Compare To Constant3/1 -> Logical Operator20/2
  Logical Operator20/1 -> RecvRStEnCtrl1/Enable
  32BitSelector16/1(y) -> Logical Operator21/1
  [IS557] -> Logical Operator21/2
  Logical Operator21/1 -> Md53StEnCtrl/Enable
  32BitSelector15/1(y) -> Logical Operator22/1
  [IS557] -> Logical Operator22/2
  Logical Operator22/1 -> Md32StEnCtrl/Enable

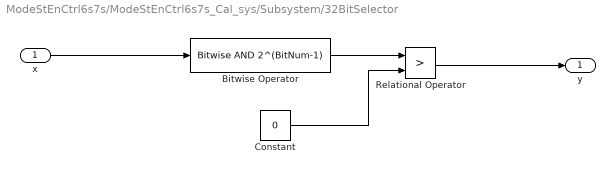
== system ModeStEnCtrl6s7s/ModeStEnCtrl6s7s_Cal_sys/Subsystem/32BitSelector ==
  x : Inport
  Bitwise Operator : simulink/Logic and Bit Operations/Bitwise Operator  logicop=AND  UseBitMask=on  BitMask=2^(BitNum-1)  BitMaskRealWorld=Stored Integer
  Constant : Constant  Value=0  OutDataTypeStr=uint32
  Relational Operator : RelationalOperator  Operator=>  OutDataTypeStr=boolean  RndMeth=Simplest  InputSameDT=off
  y : Outport  VectorParamsAs1DForOutWhenUnconnected=off
  wires:
  Relational Operator/1 -> y/1
  Constant/1 -> Relational Operator/2
  x/1 -> Bitwise Operator/1
  Bitwise Operator/1 -> Relational Operator/1

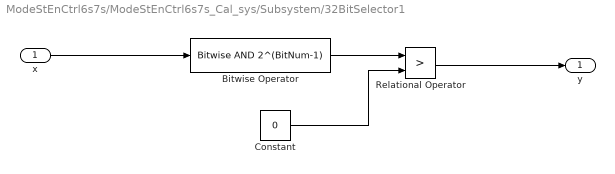
== system ModeStEnCtrl6s7s/ModeStEnCtrl6s7s_Cal_sys/Subsystem/32BitSelector1 ==
  x : Inport
  Bitwise Operator : simulink/Logic and Bit Operations/Bitwise Operator  logicop=AND  UseBitMask=on  BitMask=2^(BitNum-1)  BitMaskRealWorld=Stored Integer
  Constant : Constant  Value=0  OutDataTypeStr=uint32
  Relational Operator : RelationalOperator  Operator=>  OutDataTypeStr=boolean  RndMeth=Simplest  InputSameDT=off
  y : Outport  VectorParamsAs1DForOutWhenUnconnected=off
  wires:
  Relational Operator/1 -> y/1
  Constant/1 -> Relational Operator/2
  x/1 -> Bitwise Operator/1
  Bitwise Operator/1 -> Relational Operator/1

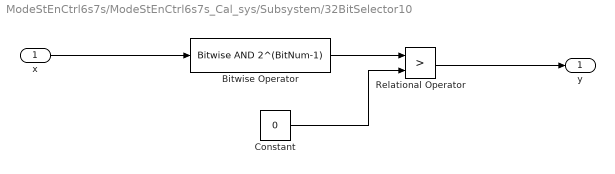
== system ModeStEnCtrl6s7s/ModeStEnCtrl6s7s_Cal_sys/Subsystem/32BitSelector10 ==
  x : Inport
  Bitwise Operator : simulink/Logic and Bit Operations/Bitwise Operator  logicop=AND  UseBitMask=on  BitMask=2^(BitNum-1)  BitMaskRealWorld=Stored Integer
  Constant : Constant  Value=0  OutDataTypeStr=uint32
  Relational Operator : RelationalOperator  Operator=>  OutDataTypeStr=boolean  RndMeth=Simplest  InputSameDT=off
  y : Outport  VectorParamsAs1DForOutWhenUnconnected=off
  wires:
  Relational Operator/1 -> y/1
  Constant/1 -> Relational Operator/2
  x/1 -> Bitwise Operator/1
  Bitwise Operator/1 -> Relational Operator/1

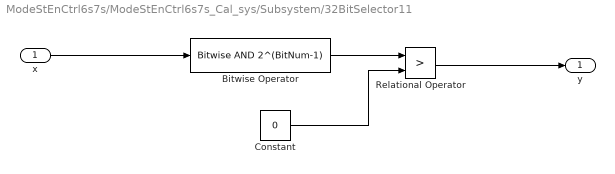
== system ModeStEnCtrl6s7s/ModeStEnCtrl6s7s_Cal_sys/Subsystem/32BitSelector11 ==
  x : Inport
  Bitwise Operator : simulink/Logic and Bit Operations/Bitwise Operator  logicop=AND  UseBitMask=on  BitMask=2^(BitNum-1)  BitMaskRealWorld=Stored Integer
  Constant : Constant  Value=0  OutDataTypeStr=uint32
  Relational Operator : RelationalOperator  Operator=>  OutDataTypeStr=boolean  RndMeth=Simplest  InputSameDT=off
  y : Outport  VectorParamsAs1DForOutWhenUnconnected=off
  wires:
  Bitwise Operator/1 -> Relational Operator/1
  x/1 -> Bitwise Operator/1
  Constant/1 -> Relational Operator/2
  Relational Operator/1 -> y/1

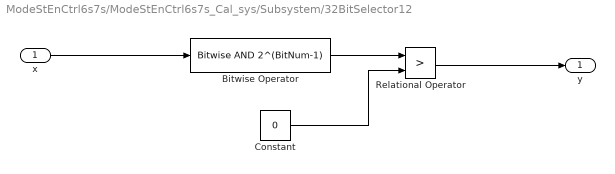
== system ModeStEnCtrl6s7s/ModeStEnCtrl6s7s_Cal_sys/Subsystem/32BitSelector12 ==
  x : Inport
  Bitwise Operator : simulink/Logic and Bit Operations/Bitwise Operator  logicop=AND  UseBitMask=on  BitMask=2^(BitNum-1)  BitMaskRealWorld=Stored Integer
  Constant : Constant  Value=0  OutDataTypeStr=uint32
  Relational Operator : RelationalOperator  Operator=>  OutDataTypeStr=boolean  RndMeth=Simplest  InputSameDT=off
  y : Outport  VectorParamsAs1DForOutWhenUnconnected=off
  wires:
  Bitwise Operator/1 -> Relational Operator/1
  x/1 -> Bitwise Operator/1
  Constant/1 -> Relational Operator/2
  Relational Operator/1 -> y/1

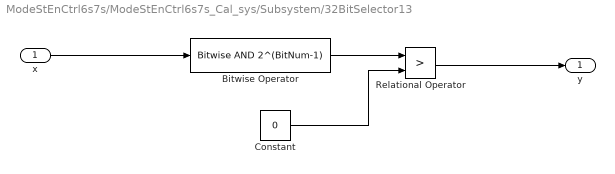
== system ModeStEnCtrl6s7s/ModeStEnCtrl6s7s_Cal_sys/Subsystem/32BitSelector13 ==
  x : Inport
  Bitwise Operator : simulink/Logic and Bit Operations/Bitwise Operator  logicop=AND  UseBitMask=on  BitMask=2^(BitNum-1)  BitMaskRealWorld=Stored Integer
  Constant : Constant  Value=0  OutDataTypeStr=uint32
  Relational Operator : RelationalOperator  Operator=>  OutDataTypeStr=boolean  RndMeth=Simplest  InputSameDT=off
  y : Outport  VectorParamsAs1DForOutWhenUnconnected=off
  wires:
  Relational Operator/1 -> y/1
  Constant/1 -> Relational Operator/2
  x/1 -> Bitwise Operator/1
  Bitwise Operator/1 -> Relational Operator/1

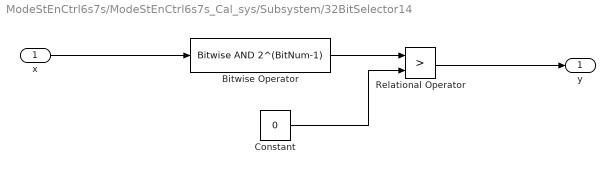
== system ModeStEnCtrl6s7s/ModeStEnCtrl6s7s_Cal_sys/Subsystem/32BitSelector14 ==
  x : Inport
  Bitwise Operator : simulink/Logic and Bit Operations/Bitwise Operator  logicop=AND  UseBitMask=on  BitMask=2^(BitNum-1)  BitMaskRealWorld=Stored Integer
  Constant : Constant  Value=0  OutDataTypeStr=uint32
  Relational Operator : RelationalOperator  Operator=>  OutDataTypeStr=boolean  RndMeth=Simplest  InputSameDT=off
  y : Outport  VectorParamsAs1DForOutWhenUnconnected=off
  wires:
  Bitwise Operator/1 -> Relational Operator/1
  x/1 -> Bitwise Operator/1
  Constant/1 -> Relational Operator/2
  Relational Operator/1 -> y/1

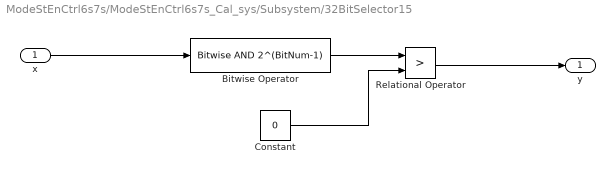
== system ModeStEnCtrl6s7s/ModeStEnCtrl6s7s_Cal_sys/Subsystem/32BitSelector15 ==
  x : Inport
  Bitwise Operator : simulink/Logic and Bit Operations/Bitwise Operator  logicop=AND  UseBitMask=on  BitMask=2^(BitNum-1)  BitMaskRealWorld=Stored Integer
  Constant : Constant  Value=0  OutDataTypeStr=uint32
  Relational Operator : RelationalOperator  Operator=>  OutDataTypeStr=boolean  RndMeth=Simplest  InputSameDT=off
  y : Outport  VectorParamsAs1DForOutWhenUnconnected=off
  wires:
  Relational Operator/1 -> y/1
  Constant/1 -> Relational Operator/2
  x/1 -> Bitwise Operator/1
  Bitwise Operator/1 -> Relational Operator/1

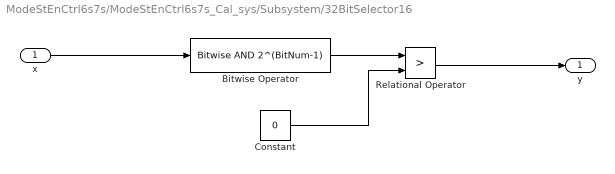
== system ModeStEnCtrl6s7s/ModeStEnCtrl6s7s_Cal_sys/Subsystem/32BitSelector16 ==
  x : Inport
  Bitwise Operator : simulink/Logic and Bit Operations/Bitwise Operator  logicop=AND  UseBitMask=on  BitMask=2^(BitNum-1)  BitMaskRealWorld=Stored Integer
  Constant : Constant  Value=0  OutDataTypeStr=uint32
  Relational Operator : RelationalOperator  Operator=>  OutDataTypeStr=boolean  RndMeth=Simplest  InputSameDT=off
  y : Outport  VectorParamsAs1DForOutWhenUnconnected=off
  wires:
  Bitwise Operator/1 -> Relational Operator/1
  x/1 -> Bitwise Operator/1
  Constant/1 -> Relational Operator/2
  Relational Operator/1 -> y/1

== system ModeStEnCtrl6s7s/ModeStEnCtrl6s7s_Cal_sys/Subsystem/32BitSelector17 ==
  x : Inport
  Bitwise Operator : simulink/Logic and Bit Operations/Bitwise Operator  logicop=AND  UseBitMask=on  BitMask=2^(BitNum-1)  BitMaskRealWorld=Stored Integer
  Constant : Constant  Value=0  OutDataTypeStr=uint32
  Relational Operator : RelationalOperator  Operator=>  OutDataTypeStr=boolean  RndMeth=Simplest  InputSameDT=off
  y : Outport  VectorParamsAs1DForOutWhenUnconnected=off
  wires:
  Relational Operator/1 -> y/1
  Constant/1 -> Relational Operator/2
  x/1 -> Bitwise Operator/1
  Bitwise Operator/1 -> Relational Operator/1

== system ModeStEnCtrl6s7s/ModeStEnCtrl6s7s_Cal_sys/Subsystem/32BitSelector18 ==
  x : Inport
  Bitwise Operator : simulink/Logic and Bit Operations/Bitwise Operator  logicop=AND  UseBitMask=on  BitMask=2^(BitNum-1)  BitMaskRealWorld=Stored Integer
  Constant : Constant  Value=0  OutDataTypeStr=uint32
  Relational Operator : RelationalOperator  Operator=>  OutDataTypeStr=boolean  RndMeth=Simplest  InputSameDT=off
  y : Outport  VectorParamsAs1DForOutWhenUnconnected=off
  wires:
  Bitwise Operator/1 -> Relational Operator/1
  x/1 -> Bitwise Operator/1
  Constant/1 -> Relational Operator/2
  Relational Operator/1 -> y/1

== system ModeStEnCtrl6s7s/ModeStEnCtrl6s7s_Cal_sys/Subsystem/32BitSelector19 ==
  x : Inport
  Bitwise Operator : simulink/Logic and Bit Operations/Bitwise Operator  logicop=AND  UseBitMask=on  BitMask=2^(BitNum-1)  BitMaskRealWorld=Stored Integer
  Constant : Constant  Value=0  OutDataTypeStr=uint32
  Relational Operator : RelationalOperator  Operator=>  OutDataTypeStr=boolean  RndMeth=Simplest  InputSameDT=off
  y : Outport  VectorParamsAs1DForOutWhenUnconnected=off
  wires:
  Bitwise Operator/1 -> Relational Operator/1
  x/1 -> Bitwise Operator/1
  Constant/1 -> Relational Operator/2
  Relational Operator/1 -> y/1

== system ModeStEnCtrl6s7s/ModeStEnCtrl6s7s_Cal_sys/Subsystem/32BitSelector2 ==
  x : Inport
  Bitwise Operator : simulink/Logic and Bit Operations/Bitwise Operator  logicop=AND  UseBitMask=on  BitMask=2^(BitNum-1)  BitMaskRealWorld=Stored Integer
  Constant : Constant  Value=0  OutDataTypeStr=uint32
  Relational Operator : RelationalOperator  Operator=>  OutDataTypeStr=boolean  RndMeth=Simplest  InputSameDT=off
  y : Outport  VectorParamsAs1DForOutWhenUnconnected=off
  wires:
  Bitwise Operator/1 -> Relational Operator/1
  x/1 -> Bitwise Operator/1
  Constant/1 -> Relational Operator/2
  Relational Operator/1 -> y/1

== system ModeStEnCtrl6s7s/ModeStEnCtrl6s7s_Cal_sys/Subsystem/32BitSelector20 ==
  x : Inport
  Bitwise Operator : simulink/Logic and Bit Operations/Bitwise Operator  logicop=AND  UseBitMask=on  BitMask=2^(BitNum-1)  BitMaskRealWorld=Stored Integer
  Constant : Constant  Value=0  OutDataTypeStr=uint32
  Relational Operator : RelationalOperator  Operator=>  OutDataTypeStr=boolean  RndMeth=Simplest  InputSameDT=off
  y : Outport  VectorParamsAs1DForOutWhenUnconnected=off
  wires:
  Relational Operator/1 -> y/1
  Constant/1 -> Relational Operator/2
  x/1 -> Bitwise Operator/1
  Bitwise Operator/1 -> Relational Operator/1

== system ModeStEnCtrl6s7s/ModeStEnCtrl6s7s_Cal_sys/Subsystem/32BitSelector21 ==
  x : Inport
  Bitwise Operator : simulink/Logic and Bit Operations/Bitwise Operator  logicop=AND  UseBitMask=on  BitMask=2^(BitNum-1)  BitMaskRealWorld=Stored Integer
  Constant : Constant  Value=0  OutDataTypeStr=uint32
  Relational Operator : RelationalOperator  Operator=>  OutDataTypeStr=boolean  RndMeth=Simplest  InputSameDT=off
  y : Outport  VectorParamsAs1DForOutWhenUnconnected=off
  wires:
  Relational Operator/1 -> y/1
  Constant/1 -> Relational Operator/2
  x/1 -> Bitwise Operator/1
  Bitwise Operator/1 -> Relational Operator/1

== system ModeStEnCtrl6s7s/ModeStEnCtrl6s7s_Cal_sys/Subsystem/32BitSelector22 ==
  x : Inport
  Bitwise Operator : simulink/Logic and Bit Operations/Bitwise Operator  logicop=AND  UseBitMask=on  BitMask=2^(BitNum-1)  BitMaskRealWorld=Stored Integer
  Constant : Constant  Value=0  OutDataTypeStr=uint32
  Relational Operator : RelationalOperator  Operator=>  OutDataTypeStr=boolean  RndMeth=Simplest  InputSameDT=off
  y : Outport  VectorParamsAs1DForOutWhenUnconnected=off
  wires:
  Bitwise Operator/1 -> Relational Operator/1
  x/1 -> Bitwise Operator/1
  Constant/1 -> Relational Operator/2
  Relational Operator/1 -> y/1

== system ModeStEnCtrl6s7s/ModeStEnCtrl6s7s_Cal_sys/Subsystem/32BitSelector23 ==
  x : Inport
  Bitwise Operator : simulink/Logic and Bit Operations/Bitwise Operator  logicop=AND  UseBitMask=on  BitMask=2^(BitNum-1)  BitMaskRealWorld=Stored Integer
  Constant : Constant  Value=0  OutDataTypeStr=uint32
  Relational Operator : RelationalOperator  Operator=>  OutDataTypeStr=boolean  RndMeth=Simplest  InputSameDT=off
  y : Outport  VectorParamsAs1DForOutWhenUnconnected=off
  wires:
  Relational Operator/1 -> y/1
  Constant/1 -> Relational Operator/2
  x/1 -> Bitwise Operator/1
  Bitwise Operator/1 -> Relational Operator/1

== system ModeStEnCtrl6s7s/ModeStEnCtrl6s7s_Cal_sys/Subsystem/32BitSelector24 ==
  x : Inport
  Bitwise Operator : simulink/Logic and Bit Operations/Bitwise Operator  logicop=AND  UseBitMask=on  BitMask=2^(BitNum-1)  BitMaskRealWorld=Stored Integer
  Constant : Constant  Value=0  OutDataTypeStr=uint32
  Relational Operator : RelationalOperator  Operator=>  OutDataTypeStr=boolean  RndMeth=Simplest  InputSameDT=off
  y : Outport  VectorParamsAs1DForOutWhenUnconnected=off
  wires:
  Relational Operator/1 -> y/1
  Constant/1 -> Relational Operator/2
  x/1 -> Bitwise Operator/1
  Bitwise Operator/1 -> Relational Operator/1

== system ModeStEnCtrl6s7s/ModeStEnCtrl6s7s_Cal_sys/Subsystem/32BitSelector25 ==
  x : Inport
  Bitwise Operator : simulink/Logic and Bit Operations/Bitwise Operator  logicop=AND  UseBitMask=on  BitMask=2^(BitNum-1)  BitMaskRealWorld=Stored Integer
  Constant : Constant  Value=0  OutDataTypeStr=uint32
  Relational Operator : RelationalOperator  Operator=>  OutDataTypeStr=boolean  RndMeth=Simplest  InputSameDT=off
  y : Outport  VectorParamsAs1DForOutWhenUnconnected=off
  wires:
  Relational Operator/1 -> y/1
  Constant/1 -> Relational Operator/2
  x/1 -> Bitwise Operator/1
  Bitwise Operator/1 -> Relational Operator/1

== system ModeStEnCtrl6s7s/ModeStEnCtrl6s7s_Cal_sys/Subsystem/32BitSelector3 ==
  x : Inport
  Bitwise Operator : simulink/Logic and Bit Operations/Bitwise Operator  logicop=AND  UseBitMask=on  BitMask=2^(BitNum-1)  BitMaskRealWorld=Stored Integer
  Constant : Constant  Value=0  OutDataTypeStr=uint32
  Relational Operator : RelationalOperator  Operator=>  OutDataTypeStr=boolean  RndMeth=Simplest  InputSameDT=off
  y : Outport  VectorParamsAs1DForOutWhenUnconnected=off
  wires:
  Bitwise Operator/1 -> Relational Operator/1
  x/1 -> Bitwise Operator/1
  Constant/1 -> Relational Operator/2
  Relational Operator/1 -> y/1

== system ModeStEnCtrl6s7s/ModeStEnCtrl6s7s_Cal_sys/Subsystem/32BitSelector4 ==
  x : Inport
  Bitwise Operator : simulink/Logic and Bit Operations/Bitwise Operator  logicop=AND  UseBitMask=on  BitMask=2^(BitNum-1)  BitMaskRealWorld=Stored Integer
  Constant : Constant  Value=0  OutDataTypeStr=uint32
  Relational Operator : RelationalOperator  Operator=>  OutDataTypeStr=boolean  RndMeth=Simplest  InputSameDT=off
  y : Outport  VectorParamsAs1DForOutWhenUnconnected=off
  wires:
  Relational Operator/1 -> y/1
  Constant/1 -> Relational Operator/2
  x/1 -> Bitwise Operator/1
  Bitwise Operator/1 -> Relational Operator/1

== system ModeStEnCtrl6s7s/ModeStEnCtrl6s7s_Cal_sys/Subsystem/32BitSelector5 ==
  x : Inport
  Bitwise Operator : simulink/Logic and Bit Operations/Bitwise Operator  logicop=AND  UseBitMask=on  BitMask=2^(BitNum-1)  BitMaskRealWorld=Stored Integer
  Constant : Constant  Value=0  OutDataTypeStr=uint32
  Relational Operator : RelationalOperator  Operator=>  OutDataTypeStr=boolean  RndMeth=Simplest  InputSameDT=off
  y : Outport  VectorParamsAs1DForOutWhenUnconnected=off
  wires:
  Bitwise Operator/1 -> Relational Operator/1
  x/1 -> Bitwise Operator/1
  Constant/1 -> Relational Operator/2
  Relational Operator/1 -> y/1

== system ModeStEnCtrl6s7s/ModeStEnCtrl6s7s_Cal_sys/Subsystem/32BitSelector6 ==
  x : Inport
  Bitwise Operator : simulink/Logic and Bit Operations/Bitwise Operator  logicop=AND  UseBitMask=on  BitMask=2^(BitNum-1)  BitMaskRealWorld=Stored Integer
  Constant : Constant  Value=0  OutDataTypeStr=uint32
  Relational Operator : RelationalOperator  Operator=>  OutDataTypeStr=boolean  RndMeth=Simplest  InputSameDT=off
  y : Outport  VectorParamsAs1DForOutWhenUnconnected=off
  wires:
  Relational Operator/1 -> y/1
  Constant/1 -> Relational Operator/2
  x/1 -> Bitwise Operator/1
  Bitwise Operator/1 -> Relational Operator/1

== system ModeStEnCtrl6s7s/ModeStEnCtrl6s7s_Cal_sys/Subsystem/32BitSelector7 ==
  x : Inport
  Bitwise Operator : simulink/Logic and Bit Operations/Bitwise Operator  logicop=AND  UseBitMask=on  BitMask=2^(BitNum-1)  BitMaskRealWorld=Stored Integer
  Constant : Constant  Value=0  OutDataTypeStr=uint32
  Relational Operator : RelationalOperator  Operator=>  OutDataTypeStr=boolean  RndMeth=Simplest  InputSameDT=off
  y : Outport  VectorParamsAs1DForOutWhenUnconnected=off
  wires:
  Bitwise Operator/1 -> Relational Operator/1
  x/1 -> Bitwise Operator/1
  Constant/1 -> Relational Operator/2
  Relational Operator/1 -> y/1

== system ModeStEnCtrl6s7s/ModeStEnCtrl6s7s_Cal_sys/Subsystem/32BitSelector8 ==
  x : Inport
  Bitwise Operator : simulink/Logic and Bit Operations/Bitwise Operator  logicop=AND  UseBitMask=on  BitMask=2^(BitNum-1)  BitMaskRealWorld=Stored Integer
  Constant : Constant  Value=0  OutDataTypeStr=uint32
  Relational Operator : RelationalOperator  Operator=>  OutDataTypeStr=boolean  RndMeth=Simplest  InputSameDT=off
  y : Outport  VectorParamsAs1DForOutWhenUnconnected=off
  wires:
  Relational Operator/1 -> y/1
  Constant/1 -> Relational Operator/2
  x/1 -> Bitwise Operator/1
  Bitwise Operator/1 -> Relational Operator/1

== system ModeStEnCtrl6s7s/ModeStEnCtrl6s7s_Cal_sys/Subsystem/32BitSelector9 ==
  x : Inport
  Bitwise Operator : simulink/Logic and Bit Operations/Bitwise Operator  logicop=AND  UseBitMask=on  BitMask=2^(BitNum-1)  BitMaskRealWorld=Stored Integer
  Constant : Constant  Value=0  OutDataTypeStr=uint32
  Relational Operator : RelationalOperator  Operator=>  OutDataTypeStr=boolean  RndMeth=Simplest  InputSameDT=off
  y : Outport  VectorParamsAs1DForOutWhenUnconnected=off
  wires:
  Relational Operator/1 -> y/1
  Constant/1 -> Relational Operator/2
  x/1 -> Bitwise Operator/1
  Bitwise Operator/1 -> Relational Operator/1
